simulink model "TPS"  (R2022b)
settings: Solver=VariableStepAuto  StartTime=0.0  StopTime=10.0  RelTol=1e-3
undefined symbols (not defined in the file): TPS_Modes
settings Model: Creator=ahmed  LastModifiedBy=ahmed
settings DebuggingCC: ParameterPrecisionLossMsg=none

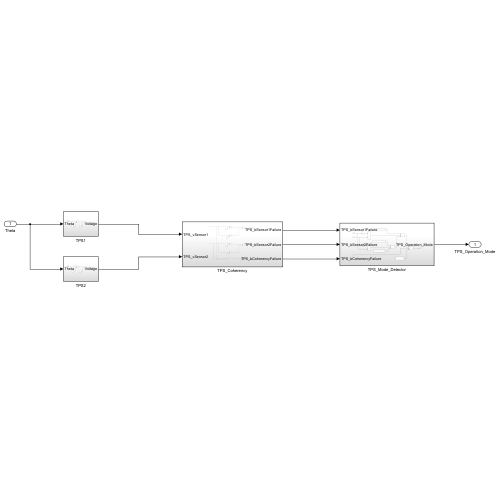
[thumbnail: Simulink's stored preview of the top-level diagram]
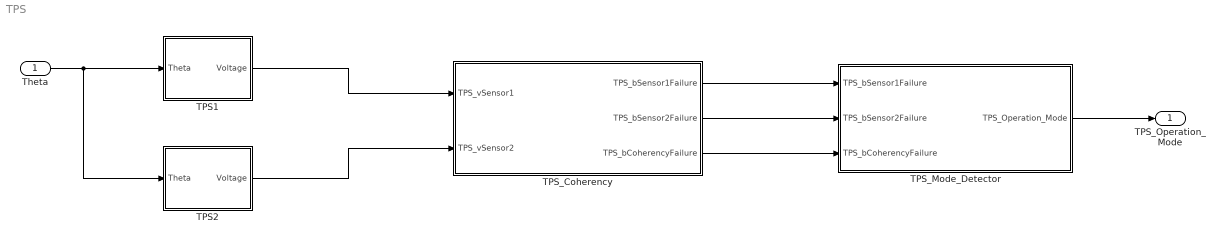
== system TPS ==
  Theta : Inport
  TPS1 : Subsystem
  TPS2 : Subsystem
  TPS_Coherency : Subsystem
  TPS_Mode_Detector : Subsystem
  TPS_Operation_Mode : Outport  OutDataTypeStr=Enum: TPS_Modes
  wires:
  Theta/1 -> TPS2/1(Theta), TPS1/1(Theta)
  TPS1/1(Voltage) -> TPS_Coherency/1(TPS_vSensor1)
  TPS2/1(Voltage) -> TPS_Coherency/2(TPS_vSensor2)
  TPS_Mode_Detector/1(TPS_Operation_Mode) -> TPS_Operation_Mode/1
  TPS_Coherency/1(TPS_bSensor1Failure) -> TPS_Mode_Detector/1(TPS_bSensor1Failure)
  TPS_Coherency/2(TPS_bSensor2Failure) -> TPS_Mode_Detector/2(TPS_bSensor2Failure)
  TPS_Coherency/3(TPS_bCoherencyFailure) -> TPS_Mode_Detector/3(TPS_bCoherencyFailure)

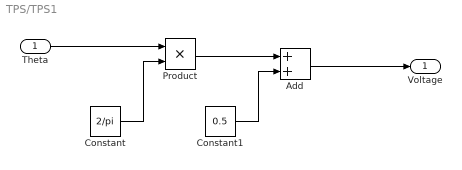
== system TPS/TPS1 ==
  Theta : Inport
  Add : Sum
  Constant : Constant  Value=2/pi  OutDataTypeStr=single
  Constant1 : Constant  Value=0.5  OutDataTypeStr=single
  Product : Product
  Voltage : Outport
  wires:
  Theta/1 -> Product/1
  Constant1/1 -> Add/2
  Add/1 -> Voltage/1
  Product/1 -> Add/1
  Constant/1 -> Product/2

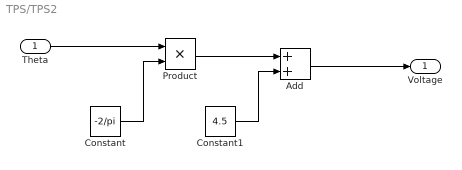
== system TPS/TPS2 ==
  Theta : Inport
  Add : Sum
  Constant : Constant  Value=-2/pi  OutDataTypeStr=single
  Constant1 : Constant  Value=4.5  OutDataTypeStr=single
  Product : Product
  Voltage : Outport  OutDataTypeStr=single
  wires:
  Constant/1 -> Product/2
  Product/1 -> Add/1
  Add/1 -> Voltage/1
  Constant1/1 -> Add/2
  Theta/1 -> Product/1

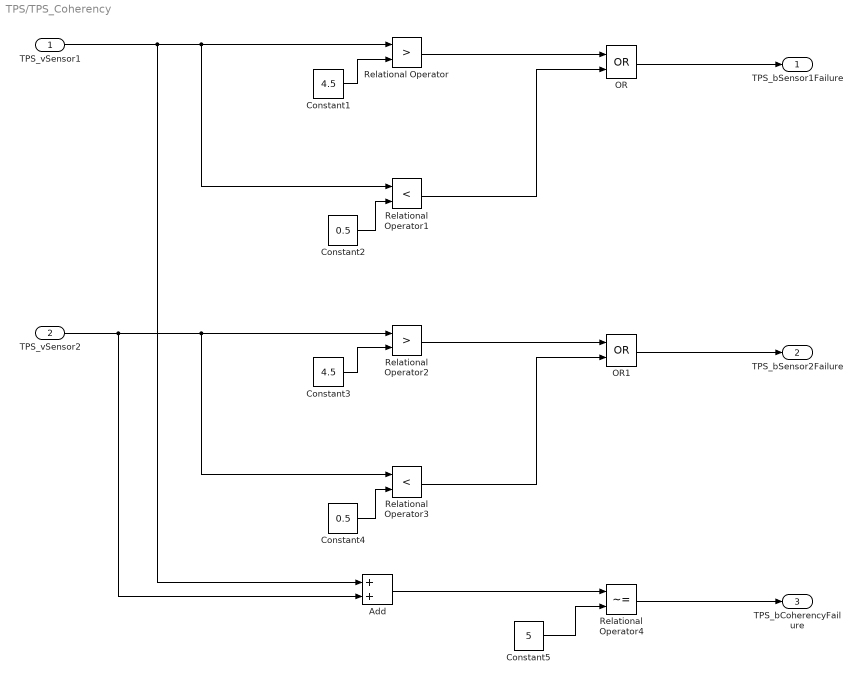
== system TPS/TPS_Coherency ==
  TPS_vSensor1 : Inport  OutDataTypeStr=single
  TPS_vSensor2 : Inport  Port=2  OutDataTypeStr=single
  Add : Sum
  Constant1 : Constant  Value=4.5
  Constant2 : Constant  Value=0.5
  Constant3 : Constant  Value=4.5
  Constant4 : Constant  Value=0.5
  Constant5 : Constant  Value=5
  OR : Logic  Operator=OR  AllPortsSameDT=off  OutDataTypeStr=boolean
  OR1 : Logic  Operator=OR  AllPortsSameDT=off  OutDataTypeStr=boolean
  Relational Operator : RelationalOperator  Operator=>  OutDataTypeStr=boolean  RndMeth=Simplest  InputSameDT=off
  Relational Operator1 : RelationalOperator  Operator=<  OutDataTypeStr=boolean  RndMeth=Simplest  InputSameDT=off
  Relational Operator2 : RelationalOperator  Operator=>  OutDataTypeStr=boolean  RndMeth=Simplest  InputSameDT=off
  Relational Operator3 : RelationalOperator  Operator=<  OutDataTypeStr=boolean  RndMeth=Simplest  InputSameDT=off
  Relational Operator4 : RelationalOperator  Operator=~=  OutDataTypeStr=boolean  RndMeth=Simplest  InputSameDT=off
  TPS_bSensor1Failure : Outport  OutDataTypeStr=boolean
  TPS_bSensor2Failure : Outport  Port=2  OutDataTypeStr=boolean
  TPS_bCoherencyFailure : Outport  Port=3  OutDataTypeStr=boolean
  wires:
  Constant2/1 -> Relational Operator1/2
  Relational Operator3/1 -> OR1/2
  Relational Operator/1 -> OR/1
  TPS_vSensor2/1 -> Relational Operator3/1, Relational Operator2/1, Add/2
  Constant4/1 -> Relational Operator3/2
  Constant1/1 -> Relational Operator/2
  Relational Operator2/1 -> OR1/1
  OR1/1 -> TPS_bSensor2Failure/1
  TPS_vSensor1/1 -> Relational Operator1/1, Relational Operator/1, Add/1
  Relational Operator4/1 -> TPS_bCoherencyFailure/1
  Constant5/1 -> Relational Operator4/2
  Add/1 -> Relational Operator4/1
  Constant3/1 -> Relational Operator2/2
  Relational Operator1/1 -> OR/2
  OR/1 -> TPS_bSensor1Failure/1

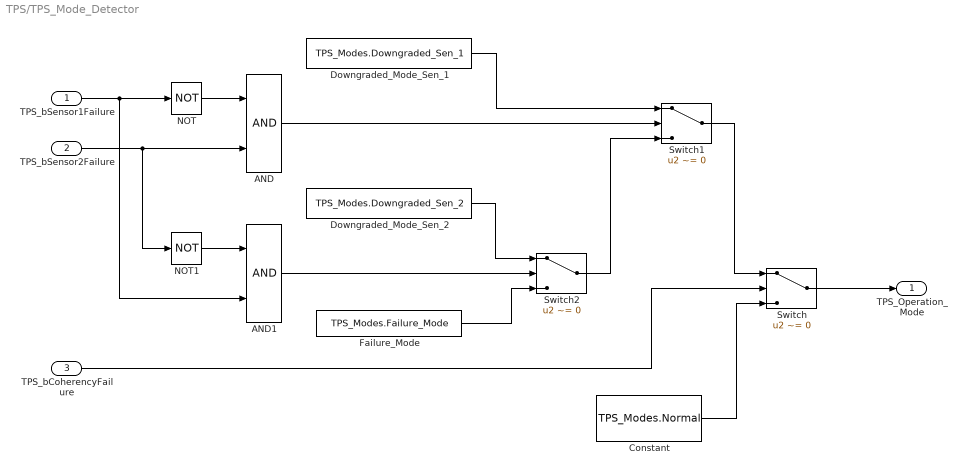
== system TPS/TPS_Mode_Detector ==
  TPS_bSensor1Failure : Inport  OutDataTypeStr=boolean
  TPS_bSensor2Failure : Inport  Port=2  OutDataTypeStr=boolean
  TPS_bCoherencyFailure : Inport  Port=3  OutDataTypeStr=boolean
  AND : Logic  AllPortsSameDT=off  OutDataTypeStr=boolean
  AND1 : Logic  AllPortsSameDT=off  OutDataTypeStr=boolean
  Constant : Constant  Value=TPS_Modes.Normal
  Downgraded_Mode_Sen_1 : Constant  Value=TPS_Modes.Downgraded_Sen_1
  Downgraded_Mode_Sen_2 : Constant  Value=TPS_Modes.Downgraded_Sen_2
  Failure_Mode : Constant  Value=TPS_Modes.Failure_Mode
  NOT : Logic  Operator=NOT  AllPortsSameDT=off  OutDataTypeStr=boolean
  NOT1 : Logic  Operator=NOT  AllPortsSameDT=off  OutDataTypeStr=boolean
  Switch : Switch  Criteria=u2 ~= 0  SaturateOnIntegerOverflow=off  InputSameDT=off
  Switch1 : Switch  Criteria=u2 ~= 0  SaturateOnIntegerOverflow=off  InputSameDT=off
  Switch2 : Switch  Criteria=u2 ~= 0  SaturateOnIntegerOverflow=off  InputSameDT=off
  TPS_Operation_Mode : Outport  OutDataTypeStr=Enum: TPS_Modes
  wires:
  TPS_bCoherencyFailure/1 -> Switch/2
  Constant/1 -> Switch/3
  TPS_bSensor1Failure/1 -> NOT/1, AND1/2
  NOT/1 -> AND/1
  TPS_bSensor2Failure/1 -> AND/2, NOT1/1
  AND/1 -> Switch1/2
  Downgraded_Mode_Sen_1/1 -> Switch1/1
  NOT1/1 -> AND1/1
  Downgraded_Mode_Sen_2/1 -> Switch2/1
  AND1/1 -> Switch2/2
  Failure_Mode/1 -> Switch2/3
  Switch2/1 -> Switch1/3
  Switch1/1 -> Switch/1
  Switch/1 -> TPS_Operation_Mode/1
